simulink library "Lib_Solve_IterNRSolverJC_EMTAT"  (R2020b)
settings: Solver=ode45  StartTime=0.0  StopTime=10.0  RelTol=1e-3  EnableMultiTasking=on
libraries: Lib_NM_JacobianCalc_TMATS x1, Lib_NM_NewtonRaphsonSolver_EMTAT x1
Description:
  | Thomas Modules
settings Model: Creator=jwchapm2  LastModifiedBy=mebell
settings DataIOCC: LimitDataPoints=on  SaveFormat=Array  ReturnWorkspaceOutputs=off
settings OptimizationCC: ExpressionDepthLimit=2147483647  LifeSpan=inf
settings DebuggingCC: UnderspecifiedInitializationDetection=Classic  MergeDetectMultiDrivingBlocksExec=none  SolverPrmCheckMsg=warning  StateNameClashWarn=warning  SFUnexpectedBacktrackingDiag=warning  SFNoUnconditionalDefaultTransitionDiag=warning  SFExecutionAtInitializationDiag=none  ArithmeticOperatorsInVariantConditions=warning
settings HardwareCC: ProdBitPerPointer=32  ProdBitPerSizeT=32  ProdBitPerPtrDiffT=32  ProdLargestAtomicFloat=None  ProdIntDivRoundTo=Undefined  ProdEndianess=Unspecified  ProdWordSize=32  ProdHWDeviceType=32-bit Generic
settings ModelReferenceCC: PropagateSignalLabelsOutOfModel=off
settings SFSimCC: SimUseLocalCustomCode=off  CustomCodeUndefinedFunction=UseInterfaceOnly
settings RTWCC: RTWUseLocalCustomCode=off
settings CodeAppCC: StateflowObjectComments=on
settings GRTTargetCC: TargetLangStandard=C89/C90 (ANSI)
settings ConfigComp: CovMetricSettings=dw  CovSaveCumulativeToWorkspaceVar=on  CovSaveSingleToWorkspaceVar=on  CovExternalEMLEnable=off

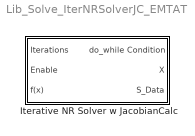
== system Lib_Solve_IterNRSolverJC_EMTAT ==
  Iterative NR Solver w JacobianCalc : Subsystem  mask(T-MATS: Iterative NR Solver w Jacobian Calc Library Block){SJac_Per_M=[0.01 0.01 0.01;-0.01 -0.01 -0.01], SNR_IC_M=[1; 2; 3], SNR_DX_M=5, SNR_Mx_M=100000, SNR_Mn_M=0.0001, SJacobianAttempts_M=20, Cond_Limits_M=0.0001}
      mask prompts: SJac_Per_M "SJac_Per_M - Jacobian Perturbation size (frac) (nxm)"; SNR_IC_M "SNR_IC_M - Newton Raphson Initial Conditions (mx1)"; SNR_DX_M "SNR_DX_M - Newton Raphson step size limiter (%) (1x1)"; SNR_Mx_M "SNR_Mx_M - Newton Raphson max limit (1x1 or mx1)"; SNR_Mn_M "SNR_Mn_M - Newton Raphson min limit (1x1 or mx1)"; SJacobianAttempts_M "SJacobianAttempts_M - Newton Raphson attempts before the Jacobian recalculation (1x1)"; Cond_Limits_M "Cond_Limits_M - Iteration Conditions Limits (mx1 or 1x1)"
      mask help:
      | The Iterative Newton Raphson Solver with Jacobian Calculator block will
      | supply the inputs to iteratively drive the outputs of a system to zero.
      |
      | This will be performed in three steps.
      | 1) Jabobian calculator sends Perturbations to the plant then calculates the plant
      | Jacboian based on the system response
      | 2) The Newton Raphson will use the inverse of the Jacobian to iteratively step the
      | system toward solution.
      | 3) Once the solution has satisfied the conditions the Newton Raphson is shut off.
      |
      | This module is designed for dynamic systems and should be paired with
      | a "do... while" block in Simulink. The "do...while" block and this module
      | should both be located in the same subsystem as the plant that is to be solved for.
      mask init:
      | if isequal(size(SNR_Mx_M),size(SNR_IC_M))
      | elseif isequal(size(SNR_Mx_M),[1 1])
      | else
      |     disp('NR_Mx_Lim_M must be the same size as NR_IC_M or a constant')
      | end
      | 
      | if isequal(size(SNR_Mn_M),size(SNR_IC_M))
      | elseif isequal(size(SNR_Mn_M),[1 1])
      | else
      |     disp('NR_Mn_Lim_M must be the same size as NR_IC_M or a constant')
      | end
      mask Help: web(which('Solver_TMATS_INRSwJC.html'),'-helpbrowser')

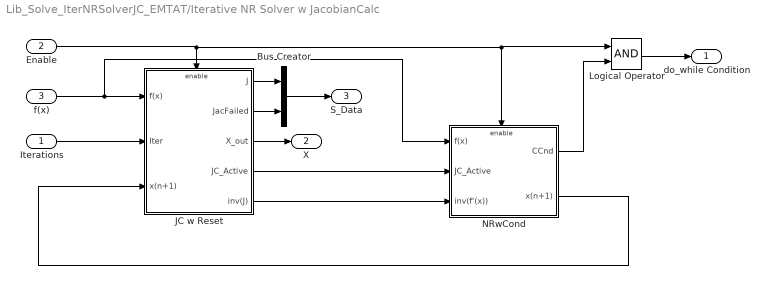
== system Lib_Solve_IterNRSolverJC_EMTAT/Iterative NR Solver w JacobianCalc ==
  Iterations : Inport  PortDimensions=1
  Enable : Inport  Port=2  PortDimensions=1
  f(x) : Inport  Port=3  PortDimensions=length(SNR_IC_M)
  Bus Creator : BusCreator  Inputs=2
  JC w Reset : Subsystem
  Logical Operator : Logic  AllPortsSameDT=off  OutDataTypeStr=boolean
  NRwCond : Subsystem
  do_while Condition : Outport  PortDimensions=1
  X : Outport  Port=2  PortDimensions=length(SNR_IC_M)
  S_Data : Outport  Port=3
  wires:
  f(x)/1 -> NRwCond/1(f(x)), JC w Reset/1(f(x))
  NRwCond/1(CCnd) -> Logical Operator/2
  Iterations/1 -> JC w Reset/2(Iter)
  NRwCond/2(x(n+1)) -> JC w Reset/3(x(n+1))
  JC w Reset/1(J) -> Bus Creator/1
  JC w Reset/3(X_out) -> X/1
  JC w Reset/4(JC_Active) -> NRwCond/2(JC_Active)
  JC w Reset/5(inv(J)) -> NRwCond/3(inv(f'(x)))
  Enable/1 -> JC w Reset/Enable, NRwCond/Enable, Logical Operator/1
  Logical Operator/1 -> do_while Condition/1
  Bus Creator/1 -> S_Data/1
  JC w Reset/2(JacFailed) -> Bus Creator/2

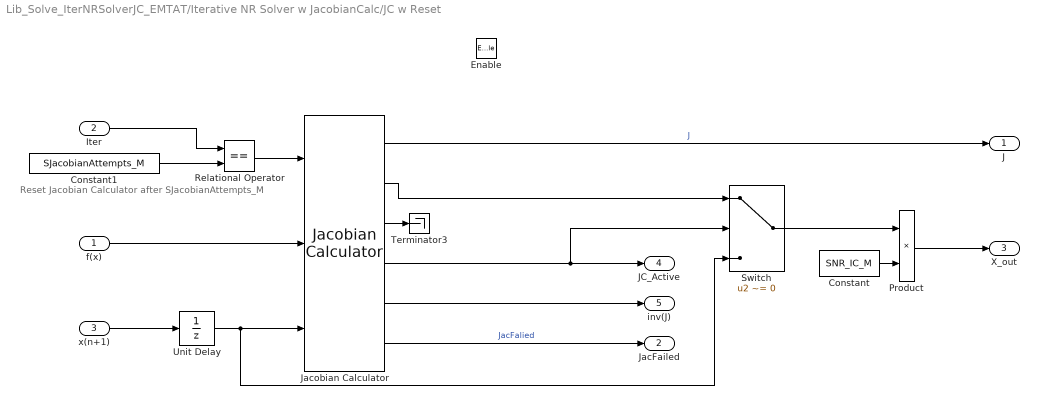
== system Lib_Solve_IterNRSolverJC_EMTAT/Iterative NR Solver w JacobianCalc/JC w Reset ==
  note: Reset Jacobian Calculator after SJacobianAttempts_M
  f(x) : Inport  PortDimensions=length(SNR_IC_M)
  Iter : Inport  Port=2  PortDimensions=1
  x(n+1) : Inport  Port=3
  Enable : EnablePort
  Constant : Constant  Value=SNR_IC_M
  Constant1 : Constant  Value=SJacobianAttempts_M  OutDataTypeStr=uint32
  Jacobian Calculator : Lib_NM_JacobianCalc_TMATS/Jacobian Calculator  N_Per_M=SJac_Per_M
  Product : Product  RndMeth=Zero
  Relational Operator : RelationalOperator  Operator===  OutDataTypeStr=boolean  RndMeth=Nearest
  Switch : Switch  Criteria=u2 ~= 0  Threshold=1
  Terminator3 : Terminator
  Unit Delay : UnitDelay  InitialCondition=ones(length(SNR_IC_M),1)  SampleTime=-1  HasFrameUpgradeWarning=on
  J : Outport  PortDimensions=[length(SNR_IC_M),length(SNR_IC_M)]
  JacFailed : Outport  Port=2  PortDimensions=1
  X_out : Outport  Port=3  PortDimensions=length(SNR_IC_M)
  JC_Active : Outport  Port=4  PortDimensions=1
  inv(J) : Outport  Port=5  PortDimensions=[length(SNR_IC_M),length(SNR_IC_M)]
  wires:
  f(x)/1 -> Jacobian Calculator/2
  Jacobian Calculator/5 -> inv(J)/1
  Unit Delay/1 -> Switch/3, Jacobian Calculator/3
  x(n+1)/1 -> Unit Delay/1
  Jacobian Calculator/1 -> J/1  "J"
  Constant/1 -> Product/2
  Relational Operator/1 -> Jacobian Calculator/1
  Product/1 -> X_out/1
  Jacobian Calculator/2 -> Switch/1
  Switch/1 -> Product/1
  Jacobian Calculator/4 -> Switch/2, JC_Active/1
  Constant1/1 -> Relational Operator/2
  Iter/1 -> Relational Operator/1
  Jacobian Calculator/3 -> Terminator3/1
  Jacobian Calculator/6 -> JacFailed/1  "JacFalied"

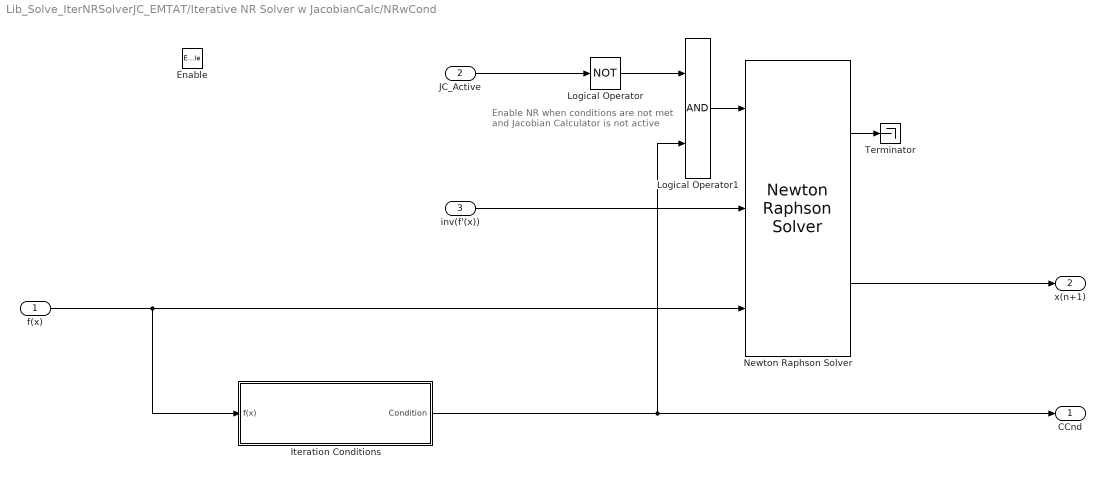
== system Lib_Solve_IterNRSolverJC_EMTAT/Iterative NR Solver w JacobianCalc/NRwCond ==
  note: Enable NR when conditions are not met
      | and Jacobian Calculator is not active
  f(x) : Inport  PortDimensions=length(SNR_IC_M)
  JC_Active : Inport  Port=2  PortDimensions=1
  inv(f'(x)) : Inport  Port=3  PortDimensions=[length(SNR_IC_M),length(SNR_IC_M)]
  Enable : EnablePort
  Iteration Conditions : Subsystem
  Logical Operator : Logic  Operator=NOT  AllPortsSameDT=off  OutDataTypeStr=boolean
  Logical Operator1 : Logic  AllPortsSameDT=off  OutDataTypeStr=boolean
  Newton Raphson Solver : Lib_NM_NewtonRaphsonSolver_EMTAT/Newton Raphson Solver  NR_IC_M=ones(size(SNR_IC_M))  NR_dx_Lim_M=SNR_DX_M  NR_Mx_Lim_M=SNR_Mx_M./SNR_IC_M  NR_Mn_Lim_M=SNR_Mn_M./SNR_IC_M  BlkNm_M=double(gcb)
  Terminator : Terminator
  CCnd : Outport  PortDimensions=1
  x(n+1) : Outport  Port=2  PortDimensions=length(SNR_IC_M)
  wires:
  f(x)/1 -> Iteration Conditions/1(f(x)), Newton Raphson Solver/3
  JC_Active/1 -> Logical Operator/1
  Newton Raphson Solver/2 -> x(n+1)/1
  Newton Raphson Solver/1 -> Terminator/1
  inv(f'(x))/1 -> Newton Raphson Solver/2
  Logical Operator1/1 -> Newton Raphson Solver/1
  Logical Operator/1 -> Logical Operator1/1
  Iteration Conditions/1(Condition) -> Logical Operator1/2, CCnd/1

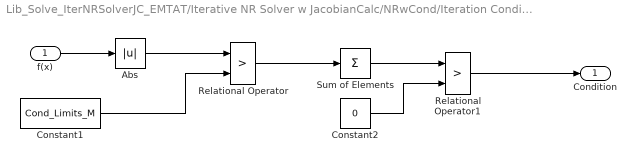
== system Lib_Solve_IterNRSolverJC_EMTAT/Iterative NR Solver w JacobianCalc/NRwCond/Iteration Conditions ==
  f(x) : Inport
  Abs : Abs
  Constant1 : Constant  Value=Cond_Limits_M
  Constant2 : Constant  Value=0
  Relational Operator : RelationalOperator  Operator=>  OutDataTypeStr=boolean  RndMeth=Nearest
  Relational Operator1 : RelationalOperator  Operator=>  OutDataTypeStr=boolean  RndMeth=Nearest
  Sum of Elements : Sum  Inputs=+
  Condition : Outport
  wires:
  Relational Operator1/1 -> Condition/1
  Sum of Elements/1 -> Relational Operator1/1
  Constant2/1 -> Relational Operator1/2
  Relational Operator/1 -> Sum of Elements/1
  f(x)/1 -> Abs/1
  Constant1/1 -> Relational Operator/2
  Abs/1 -> Relational Operator/1
